simulink model "CubeSatc"  (R2024b)
settings: Solver=ode8  StartTime=0.0  StopTime=10000  FixedStep=0.01  RelTol=1e-3
undefined symbols (not defined in the file or in its folder): env, flag, IC, orb, sat, sens
libraries: matrix_library x14
(part 3 of 3)

== system CubeSatc/Real World/Hardware Models/Sensors/Sun Sensor (Fine)/Mesurable (1) ==
  Action Port : ActionPort
  Constant : Constant
  One : Outport
  wires:
  Constant/1 -> One/1

== system CubeSatc/Real World/Hardware Models/Sensors/Sun Sensor (Fine)/Not Mesurable (0) ==
  Action Port : ActionPort
  Constant : Constant  Value=0
  Zero : Outport
  wires:
  Constant/1 -> Zero/1

== system CubeSatc/Real World/Hardware Models/Sensors/Sun Sensor (S1)/Mesurable (1) ==
  Action Port : ActionPort
  Constant : Constant
  One : Outport
  wires:
  Constant/1 -> One/1

== system CubeSatc/Real World/Hardware Models/Sensors/Sun Sensor (S1)/Not Mesurable (0) ==
  Action Port : ActionPort
  Constant : Constant  Value=0
  Zero : Outport
  wires:
  Constant/1 -> Zero/1

== system CubeSatc/Real World/Hardware Models/Sensors/Sun Sensor (S2)/Mesurable (1) ==
  Action Port : ActionPort
  Constant : Constant
  One : Outport
  wires:
  Constant/1 -> One/1

== system CubeSatc/Real World/Hardware Models/Sensors/Sun Sensor (S2)/Not Mesurable (0) ==
  Action Port : ActionPort
  Constant : Constant  Value=0
  Zero : Outport
  wires:
  Constant/1 -> Zero/1

== system CubeSatc/Real World/Hardware Models/Sensors/Sun Sensor (S3)/Mesurable (1) ==
  Action Port : ActionPort
  Constant : Constant
  One : Outport
  wires:
  Constant/1 -> One/1

== system CubeSatc/Real World/Hardware Models/Sensors/Sun Sensor (S3)/Not Mesurable (0) ==
  Action Port : ActionPort
  Constant : Constant  Value=0
  Zero : Outport
  wires:
  Constant/1 -> Zero/1

== system CubeSatc/Real World/Hardware Models/Sensors/Sun Sensor (S4)/Mesurable (1) ==
  Action Port : ActionPort
  Constant : Constant
  One : Outport
  wires:
  Constant/1 -> One/1

== system CubeSatc/Real World/Hardware Models/Sensors/Sun Sensor (S4)/Not Mesurable (0) ==
  Action Port : ActionPort
  Constant : Constant  Value=0
  Zero : Outport
  wires:
  Constant/1 -> Zero/1

== system CubeSatc/OBC/Guidance/Sun Pointing Guidance/Attitude Error/[q (-)]/Xi(q) ==
  In1 : Inport
  Demux : Demux
  Gain{,1..5} (6 alike) : Gain  Gain=-1
  Matrix Concatenate : Concatenate  NumInputs=3  Mode=Multidimensional array  ConcatenateDimension=2
  Matrix Concatenate1 : Concatenate  NumInputs=4  Mode=Multidimensional array
  Matrix Concatenate2 : Concatenate  NumInputs=4  Mode=Multidimensional array
  Matrix Concatenate3 : Concatenate  NumInputs=4  Mode=Multidimensional array
  Out1 : Outport
  wires:
  In1/1 -> Demux/1
  Demux/2 -> [q2]
  Demux/3 -> [q3]
  Demux/4 -> [q4]
  Demux/1 -> [q1]
  Matrix Concatenate/1 -> Out1/1
  Matrix Concatenate1/1 -> Matrix Concatenate/1
  Matrix Concatenate2/1 -> Matrix Concatenate/2
  Matrix Concatenate3/1 -> Matrix Concatenate/3
  Gain1/1 -> Matrix Concatenate2/4
  [q1] -> Matrix Concatenate2/3
  Gain/1 -> Matrix Concatenate1/4
  [q3] -> Matrix Concatenate1/2
  [q2] -> Matrix Concatenate3/1
  Gain5/1 -> Matrix Concatenate3/4
  [q4] -> Matrix Concatenate1/1
  [q4] -> Matrix Concatenate2/2
  [q4] -> Matrix Concatenate3/3
  [q3] -> Gain2/1
  [q3] -> Gain5/1
  [q2] -> Gain3/1
  [q2] -> Gain1/1
  [q1] -> Gain/1
  [q1] -> Gain4/1
  Gain3/1 -> Matrix Concatenate1/3
  Gain2/1 -> Matrix Concatenate2/1
  Gain4/1 -> Matrix Concatenate3/2

== system CubeSatc/Real World/DKE (Dynamics Kinematics Environment)/Environment/Perturbations/Gravity Gradient Torque/Norm ==
  Vector : Inport
  Add : Sum  Inputs=+++
  Demux : Demux  Outputs=3
  Sqrt : Sqrt
  Square : Math  Operator=square
  Square1 : Math  Operator=square
  Square2 : Math  Operator=square
  Norm : Outport
  wires:
  Square/1 -> Add/1
  Add/1 -> Sqrt/1
  Demux/3 -> Square1/1
  Square2/1 -> Add/2
  Square1/1 -> Add/3
  Demux/1 -> Square/1
  Demux/2 -> Square2/1
  Vector/1 -> Demux/1
  Sqrt/1 -> Norm/1

== system CubeSatc/Real World/DKE (Dynamics Kinematics Environment)/Environment/Perturbations/Magnetic Field Torque/Norm ==
  Vector : Inport
  Add : Sum  Inputs=+++
  Demux : Demux  Outputs=3
  Sqrt : Sqrt
  Square : Math  Operator=square
  Square1 : Math  Operator=square
  Square2 : Math  Operator=square
  Norm : Outport
  wires:
  Square/1 -> Add/1
  Add/1 -> Sqrt/1
  Demux/3 -> Square1/1
  Square2/1 -> Add/2
  Square1/1 -> Add/3
  Demux/1 -> Square/1
  Demux/2 -> Square2/1
  Vector/1 -> Demux/1
  Sqrt/1 -> Norm/1

== system CubeSatc/Real World/DKE (Dynamics Kinematics Environment)/Environment/Perturbations/Magnetic Field Torque/Norm1 ==
  Vector : Inport
  Add : Sum  Inputs=+++
  Demux : Demux  Outputs=3
  Sqrt : Sqrt
  Square : Math  Operator=square
  Square1 : Math  Operator=square
  Square2 : Math  Operator=square
  Norm : Outport
  wires:
  Square/1 -> Add/1
  Add/1 -> Sqrt/1
  Demux/3 -> Square1/1
  Square2/1 -> Add/2
  Square1/1 -> Add/3
  Demux/1 -> Square/1
  Demux/2 -> Square2/1
  Vector/1 -> Demux/1
  Sqrt/1 -> Norm/1

== system CubeSatc/Real World/DKE (Dynamics Kinematics Environment)/Environment/Perturbations/Magnetic Field Torque/Norm2 ==
  Vector : Inport
  Add : Sum  Inputs=+++
  Demux : Demux  Outputs=3
  Sqrt : Sqrt
  Square : Math  Operator=square
  Square1 : Math  Operator=square
  Square2 : Math  Operator=square
  Norm : Outport
  wires:
  Square/1 -> Add/1
  Add/1 -> Sqrt/1
  Demux/3 -> Square1/1
  Square2/1 -> Add/2
  Square1/1 -> Add/3
  Demux/1 -> Square/1
  Demux/2 -> Square2/1
  Vector/1 -> Demux/1
  Sqrt/1 -> Norm/1

== system CubeSatc/Real World/DKE (Dynamics Kinematics Environment)/Environment/Perturbations/Solar Radiation Pressure Torque/Normaliser ==
  Vector : Inport
  Constant : Constant  Value=[0; 0; 0]
  Norm1 : Subsystem
  Protected Division : Subsystem
  Switch : Switch  Criteria=u2 ~= 0  SaturateOnIntegerOverflow=off  InputSameDT=off
  Out1 : Outport
  wires:
  Norm1/1(Norm) -> Switch/2, Protected Division/2(Norm)  "norm_r"
  Switch/1 -> Out1/1
  Protected Division/1(Out1) -> Switch/1
  Vector/1 -> Protected Division/1(Vector), Norm1/1(Vector)
  Constant/1 -> Switch/3

== system CubeSatc/Real World/DKE (Dynamics Kinematics Environment)/Environment/Perturbations/Solar Radiation Pressure Torque/cross product r x F ==
  F_srp : Inport
  Constant : Constant  Value=sat.r_CM
  Matrix Concatenate{,1..3} (4 alike) : Concatenate  NumInputs=3  Mode=Multidimensional array  ConcatenateDimension=2
  Product : Product
  Product1 : Product
  Submatrix1 : matrix_library/Submatrix  RowSpan=All rows  RowStartMode=Index  RowStartIndex=1  RowEndMode=Last  RowEndIndex=1  ColSpan=One column  ColStartMode=Index  ColStartIndex=1  ColEndMode=Last  ColEndIndex=1
  Submatrix2 : matrix_library/Submatrix  RowSpan=All rows  RowStartMode=First  RowStartIndex=1  RowEndMode=Last  RowEndIndex=1  ColSpan=One column  ColStartMode=Index  ColStartIndex=2  ColEndMode=Last  ColEndIndex=1
  Submatrix3 : matrix_library/Submatrix  RowSpan=All rows  RowStartMode=Index  RowStartIndex=3  RowEndMode=Last  RowEndIndex=1  ColSpan=One column  ColStartMode=Index  ColStartIndex=3  ColEndMode=Last  ColEndIndex=1
  Submatrix6 : matrix_library/Submatrix  RowSpan=All rows  RowStartMode=Index  RowStartIndex=1  RowEndMode=Last  RowEndIndex=1  ColSpan=One column  ColStartMode=Index  ColStartIndex=1  ColEndMode=Last  ColEndIndex=1
  Submatrix7 : matrix_library/Submatrix  RowSpan=All rows  RowStartMode=First  RowStartIndex=1  RowEndMode=Last  RowEndIndex=1  ColSpan=One column  ColStartMode=Index  ColStartIndex=2  ColEndMode=Last  ColEndIndex=1
  Submatrix8 : matrix_library/Submatrix  RowSpan=All rows  RowStartMode=Index  RowStartIndex=3  RowEndMode=Last  RowEndIndex=1  ColSpan=One column  ColStartMode=Index  ColStartIndex=3  ColEndMode=Last  ColEndIndex=1
  Subtract : Sum  Inputs=+-
  Sum of Elements : Sum  Inputs=+  CollapseMode=Specified dimension
  Out1 : Outport
  wires:
  Submatrix7/1 -> Matrix Concatenate/1, Matrix Concatenate1/3
  Submatrix6/1 -> Matrix Concatenate1/2, Matrix Concatenate/3
  Submatrix8/1 -> Matrix Concatenate1/1, Matrix Concatenate/2
  Constant/1 -> Submatrix7/1, Submatrix8/1, Submatrix6/1
  Matrix Concatenate/1 -> Product/1
  Matrix Concatenate1/1 -> Product1/1
  Submatrix3/1 -> Matrix Concatenate3/1, Matrix Concatenate2/2
  Submatrix2/1 -> Matrix Concatenate3/3, Matrix Concatenate2/1
  F_srp/1 -> Submatrix2/1, Submatrix3/1, Submatrix1/1
  Submatrix1/1 -> Matrix Concatenate3/2, Matrix Concatenate2/3
  Matrix Concatenate2/1 -> Product1/2
  Matrix Concatenate3/1 -> Product/2
  Product/1 -> Subtract/1
  Product1/1 -> Subtract/2
  Subtract/1 -> Sum of Elements/1
  Sum of Elements/1 -> Out1/1

== system CubeSatc/Real World/DKE (Dynamics Kinematics Environment)/Environment/Perturbations/Solar Radiation Pressure Torque/Normaliser/Norm1 ==
  Vector : Inport
  Add : Sum  Inputs=+++
  Demux : Demux  Outputs=3
  Sqrt : Sqrt
  Square : Math  Operator=square
  Square1 : Math  Operator=square
  Square2 : Math  Operator=square
  Norm : Outport
  wires:
  Square/1 -> Add/1
  Add/1 -> Sqrt/1
  Demux/3 -> Square1/1
  Square2/1 -> Add/2
  Square1/1 -> Add/3
  Demux/1 -> Square/1
  Demux/2 -> Square2/1
  Vector/1 -> Demux/1
  Sqrt/1 -> Norm/1

== system CubeSatc/Real World/DKE (Dynamics Kinematics Environment)/Environment/Perturbations/Solar Radiation Pressure Torque/Normaliser/Protected Division ==
  Vector : Inport
  Norm : Inport  Port=2
  Constant : Constant  Value=eps
  Divide : Product  Inputs=*/
  Switch : Switch  Criteria=u2 ~= 0  SaturateOnIntegerOverflow=off  InputSameDT=off
  Out1 : Outport
  wires:
  Divide/1 -> Out1/1
  Vector/1 -> Divide/1
  Norm/1 -> Switch/1, Switch/2
  Switch/1 -> Divide/2
  Constant/1 -> Switch/3
